simulink model "AltitudeCompFilter"  (Simulink 7.8)
settings: Solver=ode45  StartTime=0.0  StopTime=10.0  RelTol=1e-3
values from neighbouring files (symbols this model uses):
  apSampleTime = 0.01    [Load_Replay.m]    (also in loadReplayMay2013.m; loadTuneRollReplay_May2013.m; replayFlight.m)
  baroCutoff = 0.2/(2*pi)    (= 0.0318309886184)    [replayFlight.m]
undefined symbols (not defined in the file or in its folder): gaind, polesd, zerosd
settings Model: Creator=User  LastModifiedBy=User

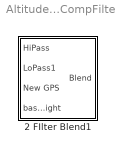
== system AltitudeCompFilter ==
  2 FIlter Blend1 : Subsystem

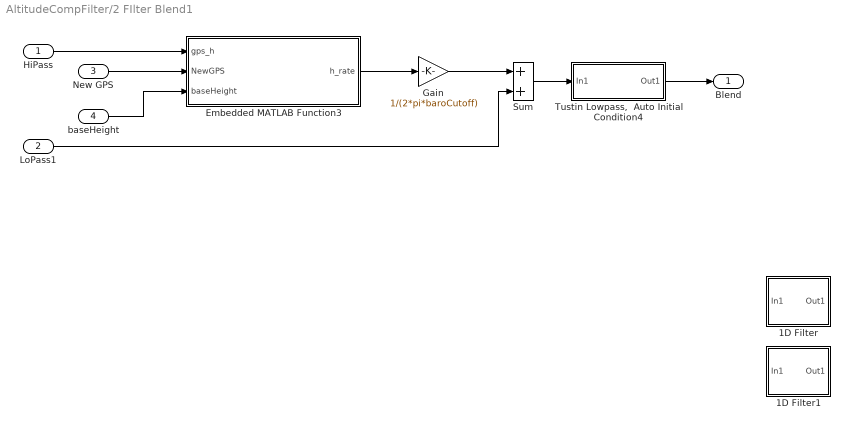
== system AltitudeCompFilter/2 FIlter Blend1 ==
  HiPass : Inport
  LoPass1 : Inport  Port=2
  New GPS : Inport  Port=3
  baseHeight : Inport  Port=4
  1D Filter : Subsystem  AncestorBlock=SLUGS_Library/Singnal Routing & Conditioning/3D Filter  RTWFcnName=TustinFilter3D  mask{zval=[], pval=-baroCutoff, kval=1, TSample=apSampleTime}
      mask prompts: zval "Zeros"; pval "Poles"; kval "Gains"; TSample "Sample Time"
      settings: RTWFcnNameOpts=User specified  RTWFileNameOpts=Use function name
      mask Display:
      | droots(zval,pval,kval)
      | port_label('input',1,'1D')
  1D Filter1 : Subsystem  AncestorBlock=SLUGS_Library/Singnal Routing & Conditioning/3D Filter  RTWFcnName=TustinFilter3D  mask{zval=[], pval=baroCutoff, kval=1, TSample=apSampleTime}
      mask prompts: zval "Zeros"; pval "Poles"; kval "Gains"; TSample "Sample Time"
      settings: RTWFcnNameOpts=User specified  RTWFileNameOpts=Use function name
      mask Display:
      | droots(zval,pval,kval)
      | port_label('input',1,'1D')
  Embedded MATLAB Function3 : MATLAB Function  TreatAsAtomicUnit=on
  Gain : Gain  Gain=1/(2*pi*baroCutoff)
  Sum : Sum  OutDataTypeStr=single
  "Tustin Lowpass,  Auto Initial Condition4" : Subsystem  mask(Tustin1stOrderLowpassAutoInitialCondition){f=baroCutoff, T=apSampleTime}
      mask prompts: f "Lowpass Frequency"; T "Sample Time"
      mask help: Takes a 3db rolloff frequency (in Hz, NOT radians/s) and a sample time. Performs a symbolic Tustin conversion and implements in a discrete filter. The initial output of the filter is set by the first sample.
      mask Help: Enter the desired 3db rolloff frequency in Hz and the sample time. Initial conditions are sampled automatically.
      mask Display: fprintf('%.2f Hz lowpass',f)
  Blend : Outport
  wires:
  Sum/1 -> "Tustin Lowpass,  Auto Initial Condition4"/1(In1)
  New GPS/1 -> Embedded MATLAB Function3/2(NewGPS)
  HiPass/1 -> Embedded MATLAB Function3/1(gps_h)
  baseHeight/1 -> Embedded MATLAB Function3/3(baseHeight)
  Embedded MATLAB Function3/1(h_rate) -> Gain/1
  "Tustin Lowpass,  Auto Initial Condition4"/1(Out1) -> Blend/1
  Gain/1 -> Sum/1
  LoPass1/1 -> Sum/2

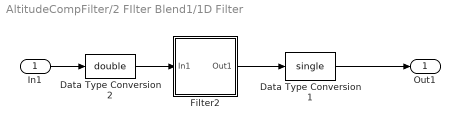
== system AltitudeCompFilter/2 FIlter Blend1/1D Filter ==
  In1 : Inport
  Data Type Conversion1 : DataTypeConversion  OutDataTypeStr=single
  Data Type Conversion2 : DataTypeConversion  OutDataTypeStr=double
  Filter2 : Subsystem  mask(DiscretizedZeroPole){Zeros=zval, Poles=pval, Gain=kval, AbsTol=auto, SampleTime=TSample, method=tustin, Wc=1}
      mask prompts: Zeros "Zeros (enter in s-main:)"; Poles "Poles (enter in s-domain:)"; Gain "Gain (enter in s-domain:)"; AbsTol "Absolute tolerance:"; SampleTime "Sample time:"; Wc "Critical Frequency (Hz):"
      mask help: Continuous mask uses c2d to transform parameters onto the Discrete Zero-Pole block inside.
      mask init:
      | st=SampleTime;
      | if length(st)>1
      |     st=SampleTime(1);
      | end
      | if(st>0)
      |     [zerosd,polesd,gaind] = sldiscutil('disczpk', {st,method,Wc,Zeros,Poles,Gain});
      | end	
      | s = get_param(gcb,'maskvalues');
      | zeross = s{1};
      | poless = s{2};
      | gainss = s{3};
      | %zerosc = eval(zeross);
      | %polesc = eval(poless);
      | %gainsc = eval(gainss);
      | sldiscutil('initzpkmask', st);
      | if(st==0)
      | set_param([gcb '/Zero Pole'], 'AbsoluteTolerance', AbsTol);
      | end
      mask StyleString: edit,edit,edit,edit,edit,popup(zoh|foh|tustin|prewarp|matched),edit
      mask CallbackString: |||||hidecrit|
      mask Display:
      | droots(zeross,poless,gainss)
      | text( 0.5, 1.0, method, 'verticalAlignment','top')
  Out1 : Outport
  wires:
  Data Type Conversion1/1 -> Out1/1
  Data Type Conversion2/1 -> Filter2/1(In1)
  In1/1 -> Data Type Conversion2/1
  Filter2/1(Out1) -> Data Type Conversion1/1

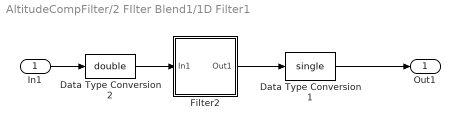
== system AltitudeCompFilter/2 FIlter Blend1/1D Filter1 ==
  In1 : Inport
  Data Type Conversion1 : DataTypeConversion  OutDataTypeStr=single
  Data Type Conversion2 : DataTypeConversion  OutDataTypeStr=double
  Filter2 : Subsystem  mask(DiscretizedZeroPole){Zeros=zval, Poles=pval, Gain=kval, AbsTol=auto, SampleTime=TSample, method=tustin, Wc=1}
      mask prompts: Zeros "Zeros (enter in s-main:)"; Poles "Poles (enter in s-domain:)"; Gain "Gain (enter in s-domain:)"; AbsTol "Absolute tolerance:"; SampleTime "Sample time:"; Wc "Critical Frequency (Hz):"
      mask help: Continuous mask uses c2d to transform parameters onto the Discrete Zero-Pole block inside.
      mask init: same as AltitudeCompFilter/2 FIlter Blend1/1D Filter/Filter2
      mask StyleString: edit,edit,edit,edit,edit,popup(zoh|foh|tustin|prewarp|matched),edit
      mask CallbackString: |||||hidecrit|
      mask Display:
      | droots(zeross,poless,gainss)
      | text( 0.5, 1.0, method, 'verticalAlignment','top')
  Out1 : Outport
  wires:
  Filter2/1(Out1) -> Data Type Conversion1/1
  In1/1 -> Data Type Conversion2/1
  Data Type Conversion2/1 -> Filter2/1(In1)
  Data Type Conversion1/1 -> Out1/1

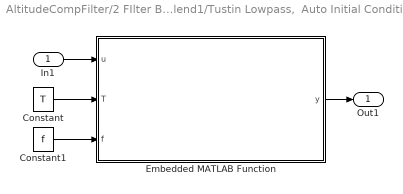
== system AltitudeCompFilter/2 FIlter Blend1/Tustin Lowpass,  Auto Initial Condition4 ==
  In1 : Inport
  Constant : Constant  Value=T
  Constant1 : Constant  Value=f
  Embedded MATLAB Function : MATLAB Function  TreatAsAtomicUnit=on
  Out1 : Outport
  wires:
  Constant/1 -> Embedded MATLAB Function/2(T)
  Constant1/1 -> Embedded MATLAB Function/3(f)
  Embedded MATLAB Function/1(y) -> Out1/1
  In1/1 -> Embedded MATLAB Function/1(u)

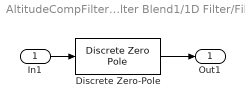
== system AltitudeCompFilter/2 FIlter Blend1/1D Filter/Filter2 ==
  In1 : Inport
  Discrete Zero-Pole : DiscreteZeroPole  Zeros=zerosd  Poles=polesd  Gain=gaind  SampleTime=SampleTime
  Out1 : Outport
  wires:
  Discrete Zero-Pole/1 -> Out1/1
  In1/1 -> Discrete Zero-Pole/1

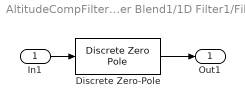
== system AltitudeCompFilter/2 FIlter Blend1/1D Filter1/Filter2 ==
  In1 : Inport
  Discrete Zero-Pole : DiscreteZeroPole  Zeros=zerosd  Poles=polesd  Gain=gaind  SampleTime=SampleTime
  Out1 : Outport
  wires:
  In1/1 -> Discrete Zero-Pole/1
  Discrete Zero-Pole/1 -> Out1/1

== matlab function 2 FIlter Blend1/Embedded MATLAB Function3 ==
  data: gps_h input double size=1; h_rate output double size=1; NewGPS input double size=1; apSampleTime parameter double size=1; baseHeight input double
function h_rate = heightRateAid(gps_h,NewGPS,apSampleTime, baseHeight)
persistent lastGps_h;
persistent TimeSinceLast;
persistent rate;
% persistent lastH;

if (isempty(lastGps_h))
    lastGps_h       = single(0.0);
    TimeSinceLast   = single(apSampleTime);
    rate            = single(0);
%     lastH           = single(-baseHeight);
%     h_rate          = single(0);
end

if (NewGPS)
    rate = single((gps_h - lastGps_h)/TimeSinceLast);
    TimeSinceLast = single(0);
    if (rate > -10.6) && (rate < 17.67)
%         h = lastH + gps_h - lastGps_h;
        h_rate = rate;
    else
%         h = lastH;
        h_rate = single(0);
    end
    lastGps_h = gps_h;
else
%     h = lastH;
    h_rate = single(0);
end

TimeSinceLast = TimeSinceLast + apSampleTime;
% lastH = h;
%%%%%%%%%%%%%%%%%%%%%%%%%%%%%%%%%%%%%%%%%%%%%%%%%%%%%%%%%%%%5
% persistent lastGps_h;
% persistent TimeSinceLast;
% persistent rate;
% persistent lastH;
% 
% if (isempty(lastGps_h))
%     lastGps_h       = single(0.0);
%     TimeSinceLast   = single(apSampleTime);
%     rate            = single(0);
%     lastH           = single(-baseHeight);
%     h_rate          = single(0);
% end
% 
% if (NewGPS)
%     rate = single((gps_h - lastGps_h)/TimeSinceLast);
%     TimeSinceLast = single(0);
%     if (rate > -10.6) && (rate < 17.67)
%         h = lastH + gps_h - lastGps_h;
% %         h_rate = rate;
%     else
%         h = lastH;
% %         h_rate = single(0);
%     end
%     lastGps_h = gps_h;
% else
%     h = lastH;
% %     h_rate = single(0);
% end
% 
% TimeSinceLast = TimeSinceLast + apSampleTime;
% lastH = h;

== matlab function 2 FIlter Blend1/Tustin Lowpass, Auto Initial Condition4/Embedded MATLAB Function ==
  data: u input double; y output double; T input double; f input double
function y = fcn(u,T,f)
% This block supports an embeddable subset of the MATLAB language.
% See the help menu for details. 

persistent a
persistent b
persistent y_km1
persistent u_km1
if isempty(a)
    %tf = [T*omega/(2+T*omega) T*omega/(2+T*omega)],[1 (T*omega-2)/(T*omega+2)]
    %tf = [a a],[1 -b]
    omega = 2*pi*f;
    a=T*omega/(2+T*omega);
    b=-(T*omega-2)/(T*omega+2);
    y_km1=u;
    u_km1=u;
end

y = a*(u+u_km1)+b*y_km1;
y_km1=y;
u_km1=u;
